simulink model "OptimisationStockageEnergy"  (R2022b)
settings: Solver=VariableStepAuto  StartTime=0.0  StopTime=1009  FixedStep=1/600  RelTol=1e-3
values from neighbouring files (symbols this model uses):
  delta_t = 0.16    [OptimisationEnergetique.m]
  PUISSANCE_Maison = elec    [OptimisationEnergetique.m]
  PV = [0 0 0 0 0 0 0 0 0 0 0 0 ... (1009 elements, 1009x1)]    [datas.mat]
  resistance = zeros(1009,1)    [OptimisationEnergetique.m]
  T_achat = 0.17/1000*6    (= 0.00102)    [OptimisationEnergetique.m]
  vec = zeros(1009,1)    [OptimisationEnergetique.m]
settings Model: Creator=33605  LastModifiedBy=33605

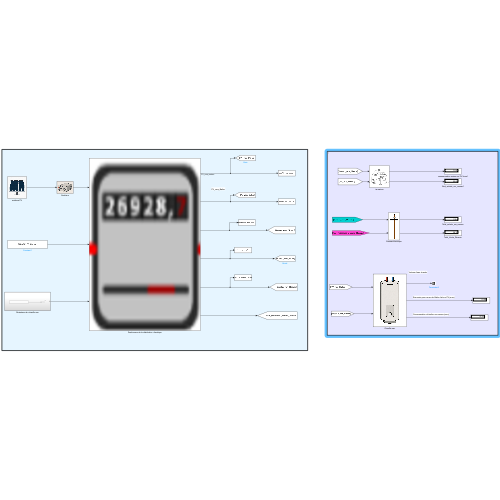
[thumbnail: Simulink's stored preview of the top-level diagram]
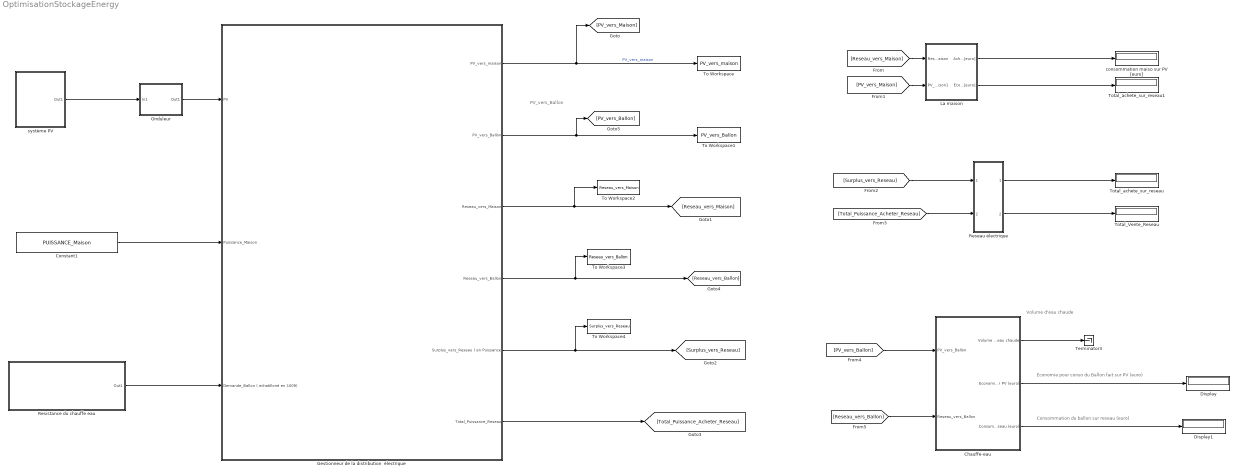
== system OptimisationStockageEnergy ==
  note: Consommation du ballon sur reseau (euro)
  note: Economie pour conso du Ballon fait sur PV (euro)
  note: PV_vers_Ballon
  note: Volume d'eau chaude
  Chauffe-eau : Subsystem
      mask Display: image('C:\Users\33605\Downloads\ChatGPT Image 5 avr. 2025, 20_55_48.png'); % Use "Edit Image" on toolstrip to change.
  Constant1 : Constant  Value=PUISSANCE_Maison
  Display : Display
  Display1 : Display
  Gestionneur de la distribution  électrique : Subsystem
      mask Display: image('C:\Users\33605\Pictures\Screenshots\Capture d''écran 2025-04-05 205904.png'); % Use "Edit Image" on toolstrip to change.
  La maison : Subsystem
      mask Display: image('C:\Users\33605\Downloads\télécharger (3).png'); % Use "Edit Image" on toolstrip to change.
  Onduleur : Subsystem
      mask Display: image('C:\Users\33605\Downloads\ChatGPT Image 5 avr. 2025, 20_50_56.png'); % Use "Edit Image" on toolstrip to change.
  Reseau électrique : Subsystem
      mask Display: image('C:\Users\33605\Downloads\Optimisation_stockage_energie-main\Optimisation_stockage_energie-main\Réseau.png'); % Use "Edit Image" on toolstrip to change.
  Resistance du chauffe eau : Subsystem
  Terminator3 : Terminator
  To Workspace : ToWorkspace  VariableName=PV_vers_maison  SaveFormat=Timeseries  SampleTime=-1
  To Workspace1 : ToWorkspace  VariableName=PV_vers_Ballon  SaveFormat=Timeseries  SampleTime=-1
  To Workspace2 : ToWorkspace  VariableName=Reseau_vers_Maison  SaveFormat=Timeseries  SampleTime=-1
  To Workspace3 : ToWorkspace  VariableName=Reseau_vers_Ballon  SaveFormat=Timeseries  SampleTime=-1
  To Workspace4 : ToWorkspace  VariableName=Surplus_vers_Reseau  SaveFormat=Timeseries  SampleTime=-1
  Total_Vente_Reseau : Display
  Total_achete_sur_reseau : Display
  Total_achete_sur_reseau1 : Display
  consommation maiso sur PV [euro] : Display
  système PV : Subsystem
      mask Display: image('C:\Users\33605\Downloads\ChatGPT Image 5 avr. 2025, 20_43_45.png'); % Use "Edit Image" on toolstrip to change.
  wires:
  Onduleur/1(Out1) -> Gestionneur de la distribution  électrique/1(PV)
  Constant1/1 -> Gestionneur de la distribution  électrique/2(Puissance_Maison)
  Resistance du chauffe eau/1(Out1) -> Gestionneur de la distribution  électrique/3(Demande_Ballon ( echatilloné en 1009))
  Gestionneur de la distribution  électrique/1(PV_vers_maison) -> [PV_vers_Maison], To Workspace/1  "PV_vers_maison"
  Gestionneur de la distribution  électrique/2(PV_vers_Ballon) -> [PV_vers_Ballon], To Workspace1/1
  Gestionneur de la distribution  électrique/3(Reseau_vers_Maison) -> To Workspace2/1, [Reseau_vers_Maison]
  Gestionneur de la distribution  électrique/4(Reseau_vers_Ballon) -> [Reseau_vers_Ballon], To Workspace3/1
  Gestionneur de la distribution  électrique/5(Surplus_vers_Reseau ( en Puissance)) -> [Surplus_vers_Reseau], To Workspace4/1
  Gestionneur de la distribution  électrique/6(Total_Puissance_Reseau) -> [Total_Puissance_Acheter_Reseau]
  système PV/1(Out1) -> Onduleur/1(In1)
  [Reseau_vers_Maison] -> La maison/1(Reseau_vers_Maison)
  La maison/1(Achat sur le réseau [euro]) -> consommation maiso sur PV [euro]/1
  [PV_vers_Maison] -> La maison/2(PV_vers_Maison1)
  La maison/2(Economie  sur PV [euro]) -> Total_achete_sur_reseau1/1
  [Total_Puissance_Acheter_Reseau] -> Reseau électrique/2(achat)
  [Surplus_vers_Reseau] -> Reseau électrique/1(surplus)
  Reseau électrique/1(Total_achete_sur_reseau) -> Total_achete_sur_reseau/1
  Reseau électrique/2(Total_vendu_sur_reseau) -> Total_Vente_Reseau/1
  Chauffe-eau/1(Volume d'eau chaude) -> Terminator3/1
  [PV_vers_Ballon] -> Chauffe-eau/1(PV_vers_Ballon)
  [Reseau_vers_Ballon] -> Chauffe-eau/2(Reseau_vers_Ballon)
  Chauffe-eau/2(Economie pour conso du Ballon fait sur PV (euro)) -> Display/1
  Chauffe-eau/3(Consommation du ballon sur reseau (euro)) -> Display1/1

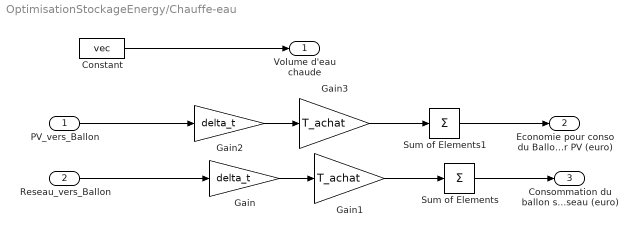
== system OptimisationStockageEnergy/Chauffe-eau ==
  PV_vers_Ballon : Inport
  Reseau_vers_Ballon : Inport  Port=2
  Constant : Constant  Value=vec
  Gain : Gain  Gain=delta_t
  Gain1 : Gain  Gain=T_achat
  Gain2 : Gain  Gain=delta_t
  Gain3 : Gain  Gain=T_achat
  Sum of Elements : Sum  Inputs=+
  Sum of Elements1 : Sum  Inputs=+
  Volume d'eau chaude : Outport
  Economie pour conso du Ballon fait sur PV (euro) : Outport  Port=2
  Consommation du ballon sur reseau (euro) : Outport  Port=3
  wires:
  Constant/1 -> Volume d'eau chaude/1
  PV_vers_Ballon/1 -> Gain2/1
  Gain1/1 -> Sum of Elements/1
  Sum of Elements/1 -> Consommation du ballon sur reseau (euro)/1
  Gain/1 -> Gain1/1
  Reseau_vers_Ballon/1 -> Gain/1
  Sum of Elements1/1 -> Economie pour conso du Ballon fait sur PV (euro)/1
  Gain2/1 -> Gain3/1
  Gain3/1 -> Sum of Elements1/1

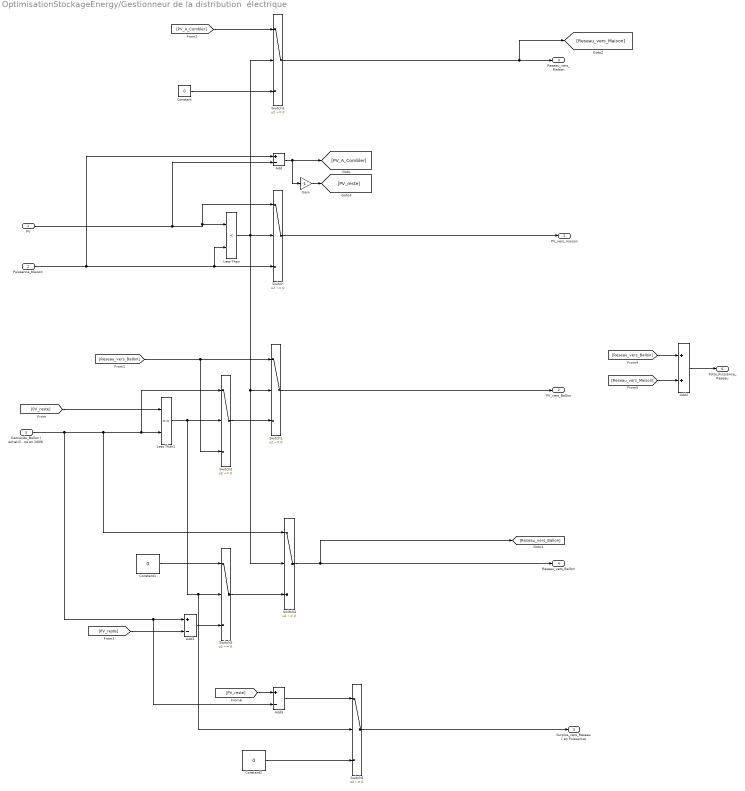
== system OptimisationStockageEnergy/Gestionneur de la distribution  électrique ==
  PV : Inport
  Puissance_Maison : Inport  Port=2
  Demande_Ballon ( echatilloné en 1009) : Inport  Port=3
  Add : Sum  Inputs=+-
  Add1 : Sum  Inputs=+-
  Add2 : Sum
  Add3 : Sum  Inputs=+-
  Constant : Constant  Value=0
  Constant1 : Constant  Value=0
  Constant2 : Constant  Value=0
  Gain : Gain  Gain=-1
  Less Than : RelationalOperator  Operator=<  OutDataTypeStr=boolean  RndMeth=Simplest  InputSameDT=off
  Less Than1 : RelationalOperator  OutDataTypeStr=boolean  RndMeth=Simplest  InputSameDT=off
  Switch{,1..6} (7 alike) : Switch  Criteria=u2 ~= 0  SaturateOnIntegerOverflow=off  InputSameDT=off
  PV_vers_maison : Outport
  PV_vers_Ballon : Outport  Port=2
  Reseau_vers_Maison : Outport  Port=3
  Reseau_vers_Ballon : Outport  Port=4
  Surplus_vers_Reseau ( en Puissance) : Outport  Port=5
  Total_Puissance_Reseau : Outport  Port=6
  wires:
  Puissance_Maison/1 -> Add/1, Less Than/2, Switch/3
  Less Than/1 -> Switch3/2, Switch/2, Switch4/2, Switch1/2
  PV/1 -> Add/2, Switch/1, Less Than/1
  Switch/1 -> PV_vers_maison/1
  [Reseau_vers_Ballon] -> Switch2/3, Switch1/1
  Switch2/1 -> Switch1/3
  Demande_Ballon ( echatilloné en 1009)/1 -> Add3/2, Add1/1, Switch4/1, Switch2/1, Less Than1/2
  Add/1 -> Gain/1, [PV_A_Combler]
  [PV_reste] -> Less Than1/1
  Less Than1/1 -> Switch6/2, Switch5/2, Switch2/2
  Switch1/1 -> PV_vers_Ballon/1
  Switch3/1 -> [Reseau_vers_Maison], Reseau_vers_Maison/1
  [PV_A_Combler] -> Switch3/1
  Constant/1 -> Switch3/3
  Switch4/1 -> [Reseau_vers_Ballon], Reseau_vers_Ballon/1
  Switch5/1 -> Switch4/3
  Constant1/1 -> Switch5/1
  Add1/1 -> Switch5/3
  [PV_reste] -> Add1/2
  [Reseau_vers_Ballon] -> Add2/1
  [Reseau_vers_Maison] -> Add2/2
  Add2/1 -> Total_Puissance_Reseau/1
  Switch6/1 -> Surplus_vers_Reseau ( en Puissance)/1
  Constant2/1 -> Switch6/3
  [PV_reste] -> Add3/1
  Add3/1 -> Switch6/1
  Gain/1 -> [PV_reste]

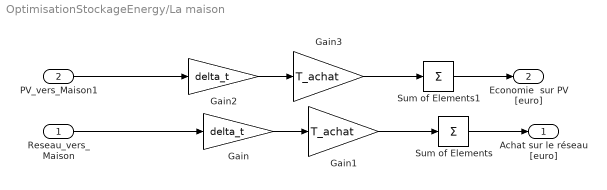
== system OptimisationStockageEnergy/La maison ==
  Reseau_vers_Maison : Inport
  PV_vers_Maison1 : Inport  Port=2
  Gain : Gain  Gain=delta_t
  Gain1 : Gain  Gain=T_achat
  Gain2 : Gain  Gain=delta_t
  Gain3 : Gain  Gain=T_achat
  Sum of Elements : Sum  Inputs=+
  Sum of Elements1 : Sum  Inputs=+
  Achat sur le réseau [euro] : Outport
  Economie  sur PV [euro] : Outport  Port=2
  wires:
  Gain/1 -> Gain1/1
  Reseau_vers_Maison/1 -> Gain/1
  Sum of Elements/1 -> Achat sur le réseau [euro]/1
  Gain1/1 -> Sum of Elements/1
  Gain3/1 -> Sum of Elements1/1
  Sum of Elements1/1 -> Economie  sur PV [euro]/1
  Gain2/1 -> Gain3/1
  PV_vers_Maison1/1 -> Gain2/1

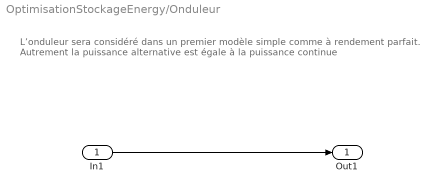
== system OptimisationStockageEnergy/Onduleur ==
  note: L’onduleur sera considéré dans un premier modèle simple comme à rendement parfait. Autrement la puissance alternative est égale à la puissance continue
  In1 : Inport
  Out1 : Outport
  wires:
  In1/1 -> Out1/1

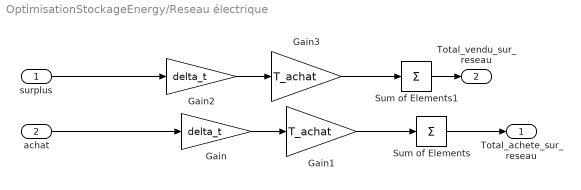
== system OptimisationStockageEnergy/Reseau électrique ==
  surplus : Inport
  achat : Inport  Port=2
  Gain : Gain  Gain=delta_t
  Gain1 : Gain  Gain=T_achat
  Gain2 : Gain  Gain=delta_t
  Gain3 : Gain  Gain=T_achat
  Sum of Elements : Sum  Inputs=+
  Sum of Elements1 : Sum  Inputs=+
  Total_achete_sur_reseau : Outport
  Total_vendu_sur_reseau : Outport  Port=2
  wires:
  surplus/1 -> Gain2/1
  Gain1/1 -> Sum of Elements/1
  Gain/1 -> Gain1/1
  achat/1 -> Gain/1
  Gain2/1 -> Gain3/1
  Gain3/1 -> Sum of Elements1/1
  Sum of Elements1/1 -> Total_vendu_sur_reseau/1
  Sum of Elements/1 -> Total_achete_sur_reseau/1

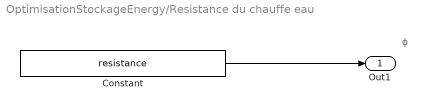
== system OptimisationStockageEnergy/Resistance du chauffe eau ==
  note: ϕ
  Constant : Constant  Value=resistance
  Out1 : Outport
  wires:
  Constant/1 -> Out1/1

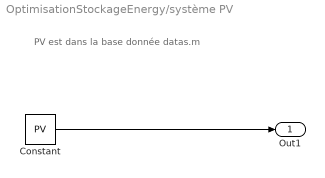
== system OptimisationStockageEnergy/système PV ==
  note: PV est dans la base donnée datas.m
  Constant : Constant  Value=PV
  Out1 : Outport
  wires:
  Constant/1 -> Out1/1
